simulink model "Airframe_Model"  (R2023b)
settings: Solver=VariableStepAuto  StartTime=0.0  StopTime=10.0  RelTol=1e-3
libraries: shared6dof x1
settings Model: Creator=plad  LastModifiedBy=plad

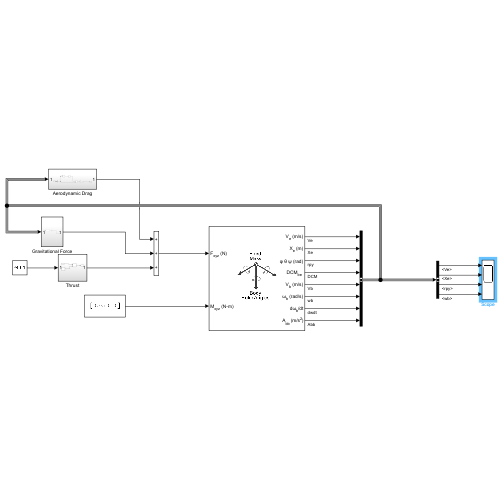
[thumbnail: Simulink's stored preview of the top-level diagram]
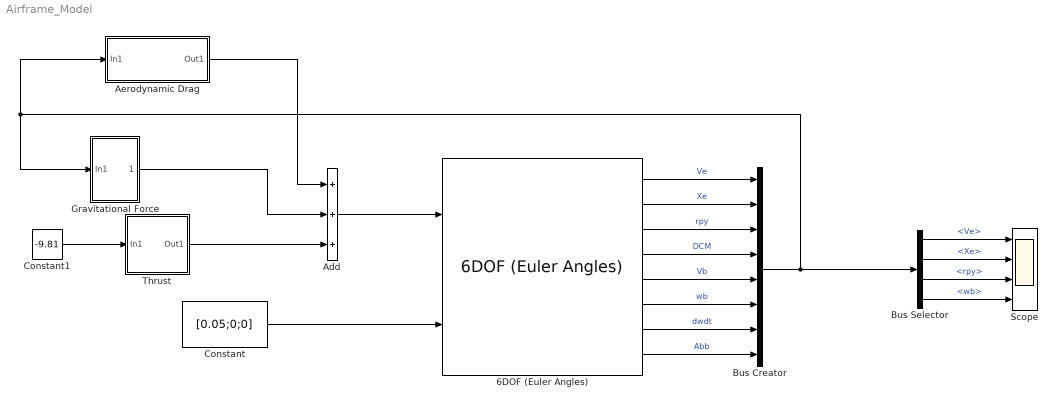
== system Airframe_Model ==
  6DOF (Euler Angles) : shared6dof/6DOF (Euler Angles)  units=Metric (MKS)  mtype=Fixed  rep=Euler Angles  xme_0=[0 0 0]  Vm_0=[0 0 0]  eul_0=[0 0 0]  pm_0=[0 0 0]  mass_0=1.0  mass_e=0.5  mass_f=2.0  inertia=eye(3)  inertia_e=eye(3)  inertia_f=2*eye(3)  k_quat=1.0  vre_flag=on  abi_flag=off  aMode=0  xme_statename=''  Vm_statename=''  eul_statename=''  quat_statename=''  pm_statename=''  mass_statename=''
  Add : Sum  Inputs=+++
  Aerodynamic Drag : Subsystem
  Bus Creator : BusCreator  Inputs=8
  Bus Selector : BusSelector  OutputSignals=Ve,Xe,rpy,wb
  Constant : Constant  Value=[0.05;0;0]
  Constant1 : Constant  Value=-9.81
  Gravitational Force : Subsystem
  Scope : Scope  NumInputPorts=4
  Thrust : Subsystem
  wires:
  6DOF (Euler Angles)/1 -> Bus Creator/1  "Ve"
  6DOF (Euler Angles)/2 -> Bus Creator/2  "Xe"
  6DOF (Euler Angles)/3 -> Bus Creator/3  "rpy"
  6DOF (Euler Angles)/4 -> Bus Creator/4  "DCM"
  6DOF (Euler Angles)/5 -> Bus Creator/5  "Vb"
  6DOF (Euler Angles)/6 -> Bus Creator/6  "wb"
  6DOF (Euler Angles)/7 -> Bus Creator/7  "dwdt"
  6DOF (Euler Angles)/8 -> Bus Creator/8  "Abb"
  Constant/1 -> 6DOF (Euler Angles)/2
  Bus Selector/2 -> Scope/2  "<Xe>"
  Bus Selector/1 -> Scope/1  "<Ve>"
  Bus Selector/3 -> Scope/3  "<rpy>"
  Bus Selector/4 -> Scope/4  "<wb>"
  Add/1 -> 6DOF (Euler Angles)/1
  Constant1/1 -> Thrust/1(In1)
  Thrust/1(Out1) -> Add/3
  Bus Creator/1 -> Aerodynamic Drag/1(In1), Gravitational Force/1(In1), Bus Selector/1
  Gravitational Force/1(Out1) -> Add/2
  Aerodynamic Drag/1(Out1) -> Add/1

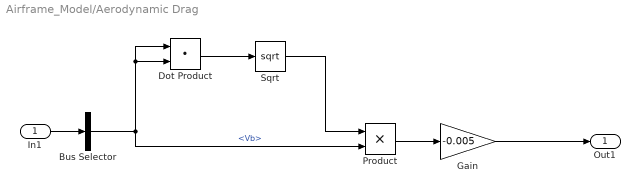
== system Airframe_Model/Aerodynamic Drag ==
  In1 : Inport
  Bus Selector : BusSelector  OutputSignals=Vb
  Dot Product : DotProduct  OutDataTypeStr=Inherit: Inherit via internal rule
  Gain : Gain  Gain=-0.005
  Product : Product
  Sqrt : Sqrt
  Out1 : Outport
  wires:
  In1/1 -> Bus Selector/1
  Bus Selector/1 -> Dot Product/1, Dot Product/2, Product/2  "<Vb>"
  Dot Product/1 -> Sqrt/1
  Sqrt/1 -> Product/1
  Product/1 -> Gain/1
  Gain/1 -> Out1/1

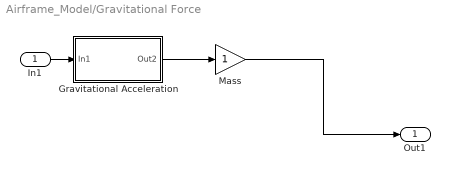
== system Airframe_Model/Gravitational Force ==
  In1 : Inport
  Gravitational Acceleration : Subsystem
  Mass : Gain
  Out1 : Outport
  wires:
  In1/1 -> Gravitational Acceleration/1(In1)
  Gravitational Acceleration/1(Out2) -> Mass/1
  Mass/1 -> Out1/1

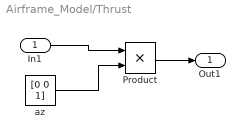
== system Airframe_Model/Thrust ==
  In1 : Inport
  Product : Product
  az : Constant  Value=[0 0 1]
  Out1 : Outport
  wires:
  az/1 -> Product/2
  Product/1 -> Out1/1
  In1/1 -> Product/1

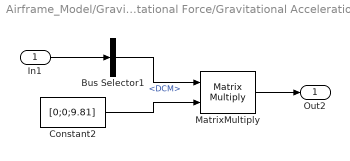
== system Airframe_Model/Gravitational Force/Gravitational Acceleration ==
  In1 : Inport
  Bus Selector1 : BusSelector  OutputSignals=DCM
  Constant2 : Constant  Value=[0;0;9.81]
  MatrixMultiply : Product  Multiplication=Matrix(*)
  Out2 : Outport
  wires:
  In1/1 -> Bus Selector1/1
  Bus Selector1/1 -> MatrixMultiply/1  "<DCM>"
  Constant2/1 -> MatrixMultiply/2
  MatrixMultiply/1 -> Out2/1
